simulink model "spherical_5th_traj_ctc"  (R2020b)
settings: Solver=ode4  StartTime=0.0  StopTime=2  FixedStep=0.001  RelTol=1e-3
values from neighbouring files (symbols this model uses):
  theta_m0_from_IK = N * theta0_from_IK    [start_taskspace_quintic_timeseries.m]
  theta_mdot0_from_IK = N * theta_dot0_from_IK    [start_taskspace_quintic_timeseries.m]
settings Model: Creator=user  LastModifiedBy=user

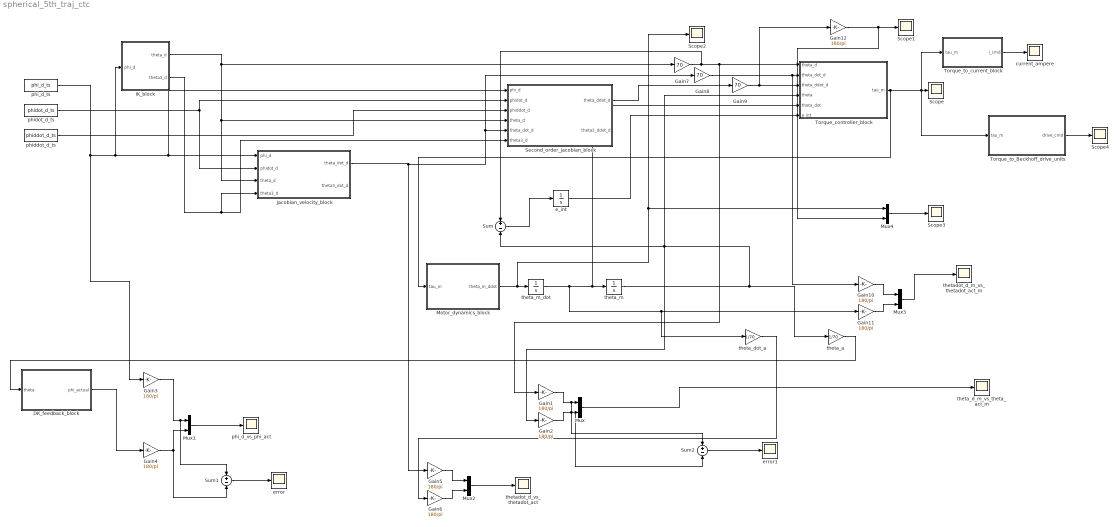
== system spherical_5th_traj_ctc ==
  DK_feedback_block : MATLAB Function  TreatAsAtomicUnit=on
  Gain{1..6,10..12} (9 alike) : Gain  Gain=180/pi
  Gain7 : Gain  Gain=70
  Gain8 : Gain  Gain=70
  Gain9 : Gain  Gain=70
  IK_block : MATLAB Function  TreatAsAtomicUnit=on
  Jacobian_velocity_block : MATLAB Function  TreatAsAtomicUnit=on
  Motor_dynamics_block : MATLAB Function  TreatAsAtomicUnit=on
  Mux{,1..4} (5 alike) : Mux  Inputs=2
  Scope{,1..4} (5 alike) : Scope
  Second_order_jacobian_block : MATLAB Function  TreatAsAtomicUnit=on
  Sum : Sum  Inputs=+-
  Sum1 : Sum  Inputs=+-
  Sum2 : Sum  Inputs=+-
  Torque_controller_block : MATLAB Function  TreatAsAtomicUnit=on
  Torque_to_Beckhoff_drive_units : MATLAB Function  TreatAsAtomicUnit=on
  Torque_to_current_block : MATLAB Function  TreatAsAtomicUnit=on
  current_ampere : Scope
  e_int : Integrator  InitialCondition=[0;0]
  error : Scope
  error1 : Scope
  phi_d_ts : FromWorkspace  VariableName=phi_d_ts  SampleTime=-1  OutputAfterFinalValue=Holding final value
  phi_d_vs_phi_act : Scope
  phiddot_d_ts : FromWorkspace  VariableName=phiddot_d_ts  SampleTime=-1  OutputAfterFinalValue=Holding final value
  phidot_d_ts : FromWorkspace  VariableName=phidot_d_ts  SampleTime=-1  OutputAfterFinalValue=Holding final value
  theta_a : Gain  Gain=1/70
  theta_d_m_vs_theta_act_m : Scope
  theta_dot_a : Gain  Gain=1/70
  theta_m : Integrator  InitialCondition=theta_m0_from_IK
  theta_m_dot : Integrator  InitialCondition=theta_mdot0_from_IK
  thetadot_d_m_vs_thetadot_act_m : Scope
  thetadot_d_vs_thetadot_act : Scope
  wires:
  phi_d_ts/1 -> Gain3/1, Jacobian_velocity_block/1(phi_d), Second_order_jacobian_block/1(phi_d), IK_block/1(phi_d)
  phidot_d_ts/1 -> Jacobian_velocity_block/2(phidot_d), Second_order_jacobian_block/2(phidot_d)
  IK_block/1(theta_d) -> Jacobian_velocity_block/3(theta_d), Second_order_jacobian_block/4(theta_d), Gain7/1
  IK_block/2(theta3_d) -> Jacobian_velocity_block/4(theta3_d), Second_order_jacobian_block/6(theta3_d)
  phiddot_d_ts/1 -> Second_order_jacobian_block/3(phiddot_d)
  Jacobian_velocity_block/1(theta_dot_d) -> Gain8/1, Second_order_jacobian_block/5(theta_dot_d), Gain5/1
  Second_order_jacobian_block/1(theta_ddot_d) -> Gain9/1
  Torque_controller_block/1(tau_m) -> Motor_dynamics_block/1(tau_m), Torque_to_current_block/1(tau_m), Scope/1, Torque_to_Beckhoff_drive_units/1(tau_m)
  Sum/1 -> e_int/1
  Mux/1 -> theta_d_m_vs_theta_act_m/1
  Gain3/1 -> Sum1/1, Mux1/1
  Mux1/1 -> phi_d_vs_phi_act/1
  Gain4/1 -> Sum1/2, Mux1/2
  DK_feedback_block/1(phi_actual) -> Gain4/1
  Gain5/1 -> Mux2/1
  Mux2/1 -> thetadot_d_vs_thetadot_act/1
  Gain6/1 -> Mux2/2
  Sum1/1 -> error/1
  Gain2/1 -> Sum2/2, Mux/2
  Sum2/1 -> error1/1
  Gain1/1 -> Sum2/1, Mux/1
  Gain7/1 -> Torque_controller_block/1(theta_d), Gain1/1, Sum/1
  Gain8/1 -> Gain10/1, Torque_controller_block/2(theta_dot_d)
  theta_m_dot/1 -> theta_m/1, Torque_controller_block/5(theta_dot), theta_dot_a/1, Gain11/1
  e_int/1 -> Torque_controller_block/6(e_int)
  theta_m/1 -> theta_a/1, Torque_controller_block/4(theta), Sum/2, Gain2/1
  theta_a/1 -> DK_feedback_block/1(theta)
  theta_dot_a/1 -> Gain6/1
  Gain11/1 -> Mux3/2
  Gain10/1 -> Mux3/1
  Mux3/1 -> thetadot_d_m_vs_thetadot_act_m/1
  Gain9/1 -> Torque_controller_block/3(theta_ddot_d), Gain12/1
  Motor_dynamics_block/1(theta_m_ddot) -> Mux4/1, Scope2/1, theta_m_dot/1
  Gain12/1 -> Mux4/2, Scope1/1
  Torque_to_current_block/1(i_cmd) -> current_ampere/1
  Mux4/1 -> Scope3/1
  Torque_to_Beckhoff_drive_units/1(drive_cmd) -> Scope4/1

== matlab function spherical_5th_traj_ctc/Jacobian_velocity_block ==
  data: phi_d input double size=[2 1]; theta_dot_d output double size=[2 1]; phidot_d input double size=[2 1]; theta_d input double size=[2 1]; theta3_d input double size=[1 1]; theta3_dot_d output double size=[1 1]
function [theta_dot_d, theta3_dot_d] = Jacobian_velocity_block(phi_d, phidot_d, theta_d, theta3_d)


deg = pi/180;

%% Robot parameters
alpha0 = pi/2;
alpha1 = pi/2;
alpha2 = pi/2;
alpha3 = pi/2;

beta1 = 0;
beta2 = 75*deg;

%% Inputs
theta1 = theta_d(1);
theta2 = theta_d(2);
theta3 = theta3_d;

phi1 = phi_d(1);

%% Rotation matrices
Rot_Y = @(a)[cos(a), 0, sin(a);
             0,      1, 0;
            -sin(a), 0, cos(a)];

Rot_DH = @(a,t)[cos(t), -sin(t)*cos(a),  sin(t)*sin(a);
                sin(t),  cos(t)*cos(a), -cos(t)*sin(a);
                0,       sin(a),         cos(a)];

%% Unit vectors
e1 = [0;0;1];
e2 = [1;0;0];

e33 = [0;0;1];
e44 = [0;0;1];
e55 = [0;0;1];

%% End-effector vector in frame 5
v5 = [sin(beta2);
      sin(beta1)*cos(beta2);
      cos(beta1)*cos(beta2)];

v5 = v5 / norm(v5);

%% Transformations
Q0 = Rot_Y(alpha0);
Q1 = Rot_DH(alpha1, theta1);
Q2 = Rot_DH(alpha2, theta2);
Q3 = Rot_DH(alpha3, theta3);

%% Vectors in frame 1
e3 = Q1 * e33;
e4 = Q0 * Q2 * e44;

e5 = Q1 * Q3 * e55;
e5 = e5 / norm(e5);

v1 = Q1 * Q3 * v5;
v1 = v1 / norm(v1);

%% Angular velocity mapping
% omega_1 = S * phidot
S = [0,  sin(phi1);
     0, -cos(phi1);
     1,  0];

%% Jacobian terms
k11 = dot(v1, cross(e1, e3));
k22 = dot(e5, cross(e2, e4));

J0 = [cross(e3, v1).';
      cross(e4, e5).'];

J = J0 * S;

%% Avoid division by exact zero
epsK = 1e-8;

if abs(k11) < epsK
    k11 = sign_or_one(k11) * epsK;
end

if abs(k22) < epsK
    k22 = sign_or_one(k22) * epsK;
end

%% Velocity mapping
% K * theta_dot = J * phi_dot
theta1_dot = (J(1,:) * phidot_d) / k11;
theta2_dot = (J(2,:) * phidot_d) / k22;

theta_dot_d = [theta1_dot;
               theta2_dot];

%% Passive joint velocity
omega = S * phidot_d;

theta3_dot_d = dot(e3, omega);

end

function y = sign_or_one(x)

if x >= 0
    y = 1;
else
    y = -1;
end

end

== matlab function spherical_5th_traj_ctc/IK_block ==
  settings: updateMethod=DISCRETE
  data: phi_d input double size=[2 1]; theta_d output double size=[2 1]; theta3_d output double size=[1 1]
function [theta_d, theta3_d] = IK_block(phi_d)


deg = pi/180;

alpha0 = pi/2;
alpha1 = pi/2;
alpha2 = pi/2;
alpha3 = pi/2;
alpha4 = pi/2;

beta1 = 0;
beta2 = 75*deg;

theta3_ref = 15*deg;

tol = 1e-9;
tolPhi1 = 1e-8;

phi1 = phi_d(1);
phi2 = phi_d(2);

d_des = direction_from_orientation(phi1, phi2);

persistent theta_prev initialized

if isempty(initialized)
    theta_prev = [0; 0; theta3_ref];
    initialized = true;
end

sols = zeros(6,3);
valid = false(6,1);
idx = 0;

%% Special DK-consistent branch
% phi1 = 0 -> theta1 = 0, theta2 = phi2, theta3 = 15 + theta2

if abs(phi1) < tolPhi1

    theta1 = 0;
    theta2 = phi2;
    theta3 = theta3_ref + theta2;

    d_check = FK_direction(theta1, theta3, beta1, beta2, alpha1, alpha3);
    err = norm(d_check - d_des);

    if err < 1e-6
        idx = idx + 1;
        sols(idx,:) = [theta1, theta2, theta3];
        valid(idx) = true;
    end
end

%% Normal IK branches

Rot_Y = @(a)[cos(a) 0 sin(a);
             0      1 0;
            -sin(a) 0 cos(a)];

Rot_DH = @(a,t)[cos(t), -sin(t)*cos(a),  sin(t)*sin(a);
                sin(t),  cos(t)*cos(a), -cos(t)*sin(a);
                0,       sin(a),         cos(a)];

Q0 = Rot_Y(alpha0);

e11 = [0;0;1];
e44 = [0;0;1];

v5 = [sin(beta2);
      sin(beta1)*cos(beta2);
      cos(beta1)*cos(beta2)];

v5 = v5 / norm(v5);

v = [ d_des(2);
     -d_des(1);
      d_des(3)];

v = v / norm(v);

vx = v(1);
vy = v(2);

b = sin(beta1)*cos(beta2);
R = sqrt(vx^2 + vy^2);

if R > tol && abs(b) <= R + tol

    ratio = clamp(b/R, -1, 1);
    psi = atan2(vy, vx);

    theta1_list = zeros(2,1);
    theta1_list(1) = wrapToPiLocal(psi + asin(ratio));
    theta1_list(2) = wrapToPiLocal(psi + pi - asin(ratio));

    a = sin(beta2);
    c = cos(beta1)*cos(beta2);

    for i = 1:2

        theta1 = theta1_list(i);
        Q1 = Rot_DH(alpha1, theta1);

        A = Q1.' * v;

        denom = a^2 + c^2;

        if denom > tol

            cos3 = (a*A(1) - c*A(2)) / denom;
            sin3 = (c*A(1) + a*A(2)) / denom;

            cos3 = clamp(cos3, -1, 1);
            sin3 = clamp(sin3, -1, 1);

            theta3 = wrapToPiLocal(atan2(sin3, cos3));
            Q3 = Rot_DH(alpha3, theta3);

            if norm(Q1*Q3*v5 - v) < 1e-6

                u = Q1 * Q3 * e11;
                u = u / norm(u);

                C = cos(alpha4);

                A2 = -u(3);
                B2 = -u(2);

                R2 = sqrt(A2^2 + B2^2);

                if R2 > tol && abs(C) <= R2 + tol

                    ratio2 = clamp(C/R2, -1, 1);
                    delta = atan2(B2, A2);

                    theta2_a = wrapToPiLocal(asin(ratio2) - delta);
                    theta2_b = wrapToPiLocal(pi - asin(ratio2) - delta);

                    theta2_list = [theta2_a; theta2_b];

                    for m = 1:2

                        theta2 = theta2_list(m);
                        Q2 = Rot_DH(alpha2, theta2);

                        e41 = Q0 * Q2 * e44;

                        constraint_error = dot(u,e41) - cos(alpha4);

                        if abs(constraint_error) < 1e-6

                            d_check = FK_direction(theta1, theta3, beta1, beta2, alpha1, alpha3);
                            err = norm(d_check - d_des);

                            if err < 1e-6 && idx < 6
                                idx = idx + 1;
                                sols(idx,:) = [theta1, theta2, theta3];
                                valid(idx) = true;
                            end
                        end
                    end
                end
            end
        end
    end
end

%% Choose solution closest to previous joint state

bestCost = 1e9;
bestTheta = theta_prev;

for k = 1:6

    if valid(k)

        theta_k = sols(k,:).';

        cost = norm(wrapToPiVec(theta_k - theta_prev));

        if cost < bestCost
            bestCost = cost;
            bestTheta = theta_k;
        end
    end
end

theta_prev = bestTheta;

theta_d = [bestTheta(1); bestTheta(2)];
theta3_d = bestTheta(3);

end

%% ============================================================
% LOCAL FUNCTIONS
%% ============================================================

function d = direction_from_orientation(phi1, phi2)

d = [-cos(phi2)*sin(phi1);
      cos(phi2)*cos(phi1);
      sin(phi2)];

d = d / norm(d);
end

function d = FK_direction(theta1, theta3, beta1, beta2, alpha1, alpha3)

Rot_DH = @(a,t)[cos(t), -sin(t)*cos(a),  sin(t)*sin(a);
                sin(t),  cos(t)*cos(a), -cos(t)*sin(a);
                0,       sin(a),         cos(a)];

Q1 = Rot_DH(alpha1, theta1);
Q3 = Rot_DH(alpha3, theta3);

v5 = [sin(beta2);
      sin(beta1)*cos(beta2);
      cos(beta1)*cos(beta2)];

v5 = v5 / norm(v5);

v1 = Q1 * Q3 * v5;
v1 = v1 / norm(v1);

d = [-v1(2);
      v1(1);
      v1(3)];

d = d / norm(d);
end

function x = clamp(x, lo, hi)

x = min(max(x, lo), hi);
end

function a = wrapToPiLocal(a)

a = atan2(sin(a), cos(a));
end

function y = wrapToPiVec(x)

y = zeros(size(x));

for i = 1:length(x)
    y(i) = atan2(sin(x(i)), cos(x(i)));
end
end

== matlab function spherical_5th_traj_ctc/Second_order_jacobian_block ==
  data: phi_d input double size=[2 1]; theta_ddot_d output double size=[2 1]; phidot_d input double size=[2 1]; phiddot_d input double size=[2 1]; theta_d input double size=[2 1]; theta_dot_d input double size=[2 1]; theta3_d input double size=[1 1]; theta3_ddot_d output double size=[1 1]
function [theta_ddot_d, theta3_ddot_d] = Second_order_jacobian_block(phi_d, phidot_d, phiddot_d, theta_d, theta_dot_d, theta3_d)


deg = pi/180;

alpha0 = pi/2;
alpha1 = pi/2;
alpha2 = pi/2;
alpha3 = pi/2;

beta1 = 0;
beta2 = 75*deg;

theta1 = theta_d(1);
theta2 = theta_d(2);
theta3 = theta3_d;

theta1_dot = theta_dot_d(1);
theta2_dot = theta_dot_d(2);

phi1 = phi_d(1);

Rot_Y = @(a)[cos(a), 0, sin(a);
             0,      1, 0;
            -sin(a), 0, cos(a)];

Rot_DH = @(a,t)[cos(t), -sin(t)*cos(a),  sin(t)*sin(a);
                sin(t),  cos(t)*cos(a), -cos(t)*sin(a);
                0,       sin(a),         cos(a)];

e1 = [0;0;1];
e2 = [1;0;0];

e33 = [0;0;1];
e44 = [0;0;1];
e55 = [0;0;1];

v5 = [sin(beta2);
      sin(beta1)*cos(beta2);
      cos(beta1)*cos(beta2)];

v5 = v5 / norm(v5);

Q0 = Rot_Y(alpha0);
Q1 = Rot_DH(alpha1, theta1);
Q2 = Rot_DH(alpha2, theta2);
Q3 = Rot_DH(alpha3, theta3);

e3 = Q1 * e33;

e4 = Q0 * Q2 * e44;

e5 = Q1 * Q3 * e55;
e5 = e5 / norm(e5);

v1 = Q1 * Q3 * v5;
v1 = v1 / norm(v1);


S = [0,  sin(phi1);
     0, -cos(phi1);
     1,  0];

Sdot = [0,  cos(phi1)*phidot_d(1);
        0,  sin(phi1)*phidot_d(1);
        0,  0];

omega = S * phidot_d;

omega_dot = S * phiddot_d + Sdot * phidot_d;


e3_dot = theta1_dot * cross(e1, e3);

e4_dot = theta2_dot * cross(e2, e4);

v1_dot = cross(omega, v1);

e5_dot = cross(omega, e5);

% e3_ddot = theta1_ddot*(e1 x e3) + theta1_dot*(e1 x e3_dot)
e3_ddot_known = theta1_dot * cross(e1, e3_dot);

% e4_ddot = theta2_ddot*(e2 x e4) + theta2_dot*(e2 x e4_dot)
e4_ddot_known = theta2_dot * cross(e2, e4_dot);

% v1_ddot = omega_dot x v1 + omega x v1_dot
v1_ddot = cross(omega_dot, v1) + cross(omega, v1_dot);

% e5_ddot = omega_dot x e5 + omega x e5_dot
e5_ddot = cross(omega_dot, e5) + cross(omega, e5_dot);

%% ============================================================
% Acceleration constraint 1
%% ============================================================
%
% C1 = e3 . v1 = constant
%
% C1_ddot =
% e3_ddot . v1 + 2 e3_dot . v1_dot + e3 . v1_ddot = 0
%
% Solve for theta1_ddot

den1 = dot(v1, cross(e1, e3));

num1 = dot(e3_ddot_known, v1) + 2 * dot(e3_dot, v1_dot)+ dot(e3, v1_ddot);

epsD = 1e-8;

if abs(den1) < epsD
    den1 = sign_or_one(den1) * epsD;
end

theta1_ddot = -num1 / den1;

%% ============================================================
% Acceleration constraint 2
%% ============================================================
%
% C2 = e4 . e5 = constant
%
% C2_ddot =
% e4_ddot . e5 + 2 e4_dot . e5_dot + e4 . e5_ddot = 0
%
% Solve for theta2_ddot

den2 = dot(e5, cross(e2, e4));

num2 = dot(e4_ddot_known, e5) + 2 * dot(e4_dot, e5_dot)+ dot(e4, e5_ddot);

if abs(den2) < epsD
    den2 = sign_or_one(den2) * epsD;
end

theta2_ddot = -num2 / den2;

theta_ddot_d = [theta1_ddot;
                theta2_ddot];

%% ============================================================
% Passive joint acceleration
%% ============================================================
%
% omega_dot = theta1_ddot*e1 + theta3_ddot*e3 + theta3_dot*e3_dot
%
% We approximate from platform angular acceleration:
%
% theta3_ddot = e3 . omega_dot

theta3_ddot_d = dot(e3, omega_dot);

end

function y = sign_or_one(x)

if x >= 0
    y = 1;
else
    y = -1;
end

end

== matlab function spherical_5th_traj_ctc/Torque_controller_block ==
  data: theta_d input double size=[2 1]; tau_m output double size=[2 1]; theta_dot_d input double size=[2 1]; theta_ddot_d input double size=[2 1]; theta input double size=[2 1]; theta_dot input double size=[2 1]; e_int input double size=[2 1]
function tau_m = Torque_controller_block(theta_d, theta_dot_d, theta_ddot_d, theta, theta_dot, e_int)

J1 = 62e-6;
J2 = 62e-6;    

%% Controller gains from Beckhoff parameter file

Wc_B = 150.0;
Wn_B = 2*Wc_B;

Ki_B = Wn_B^3;
Kp_B = 3*Wn_B^2;
Kv_B = 3*Wn_B;

Kp1 = Kp_B;
Kp2 = Kp_B;

Kd1 = Kv_B;
Kd2 = Kv_B;

Ki1 = Ki_B;
Ki2 = Ki_B;


e1 = theta_d(1) - theta(1);
e2 = theta_d(2) - theta(2);

ed1 = theta_dot_d(1) - theta_dot(1);
ed2 = theta_dot_d(2) - theta_dot(2);

ei1 = e_int(1);
ei2 = e_int(2);


v1 = theta_ddot_d(1) + Kd1*ed1 + Kp1*e1 + Ki1*ei1;
v2 = theta_ddot_d(2) + Kd2*ed2 + Kp2*e2 + Ki2*ei2;

tau1 = J1 * v1;
tau2 = J2 * v2;

%% Torque saturation
tau_max = 1.0;    % Nm

if tau1 > tau_max
    tau1 = tau_max;
elseif tau1 < -tau_max
    tau1 = -tau_max;
end

if tau2 > tau_max
    tau2 = tau_max;
elseif tau2 < -tau_max
    tau2 = -tau_max;
end

tau_m = [tau1;
       tau2];

end

== matlab function spherical_5th_traj_ctc/DK_feedback_block ==
  data: theta input double size=[2 1]; phi_actual output double size=[2 1]
function phi_actual = DK_feedback_block(theta)

deg = pi/180;

%% Robot parameters
alpha0 = pi/2;
alpha1 = pi/2;
alpha2 = pi/2;
alpha3 = pi/2;

beta1 = 0;
beta2 = 75*deg;

theta3_home = 15*deg;

tolTheta  = 1e-10;
tolTheta1 = 1e-8;
tolCross  = 1e-10;

theta1 = theta(1);
theta2 = theta(2);

%% Rotation matrices
Rot_Y = @(a)[cos(a), 0, sin(a);
             0,      1, 0;
            -sin(a), 0, cos(a)];

Rot_DH = @(a,t)[cos(t), -sin(t)*cos(a),  sin(t)*sin(a);
                sin(t),  cos(t)*cos(a), -cos(t)*sin(a);
                0,       sin(a),         cos(a)];

%% Unit vectors
e33 = [0;0;1];
e44 = [0;0;1];
e55 = [0;0;1];

%% v5
v5 = [sin(beta2);
      sin(beta1)*cos(beta2);
      cos(beta1)*cos(beta2)];

v5 = v5 / norm(v5);

%% Transformations
Q0 = Rot_Y(alpha0);
Q1 = Rot_DH(alpha1, theta1);
Q2 = Rot_DH(alpha2, theta2);

e3 = Q1 * e33;
e4 = Q0 * Q2 * e44;

cross_e = cross(e3, e4);
cross_norm = norm(cross_e);

%% DK branch logic
if abs(theta1) < tolTheta1

    % Physical theta1 = 0 branch
    theta3 = theta3_home + theta2;

elseif cross_norm < tolCross

    % Fallback at true cross-product singularity
    theta3 = theta3_home;

else

    % General DK branch
    u_plus  =  cross_e / cross_norm;
    u_minus = -cross_e / cross_norm;

    theta3_plus  = theta3_from_u(u_plus,  theta1, tolTheta);
    theta3_minus = theta3_from_u(u_minus, theta1, tolTheta);

    err_plus  = abs(wrapToPiLocal(theta3_plus  - theta3_home));
    err_minus = abs(wrapToPiLocal(theta3_minus - theta3_home));

    if err_plus <= err_minus
        theta3 = theta3_plus;
    else
        theta3 = theta3_minus;
    end
end

%% Output direction
Q3 = Rot_DH(alpha3, theta3);

v1 = Q1 * Q3 * v5;
v1 = v1 / norm(v1);

d = [-v1(2);
      v1(1);
      v1(3)];

d = d / norm(d);

phi1 = atan2(-d(1), d(2));
phi2 = asin(clamp(d(3), -1, 1));

phi_actual = [phi1;
              phi2];

end

%% ============================================================
% Helper functions
%% ============================================================

function theta3 = theta3_from_u(u, theta1, tol)

ux = u(1);
uy = u(2);
uz = u(3);

if abs(cos(theta1)) > abs(sin(theta1))
    sin_theta3 = ux / cos(theta1);
else
    if abs(sin(theta1)) < tol
        sin_theta3 = 0;
    else
        sin_theta3 = uy / sin(theta1);
    end
end

cos_theta3 = -uz;

sin_theta3 = clamp(sin_theta3, -1, 1);
cos_theta3 = clamp(cos_theta3, -1, 1);

theta3 = atan2(sin_theta3, cos_theta3);

end

function x = clamp(x, lo, hi)

x = min(max(x, lo), hi);

end

function a = wrapToPiLocal(a)

a = atan2(sin(a), cos(a));

end

== matlab function spherical_5th_traj_ctc/Motor_dynamics_block ==
  data: tau_m input double size=[2 1]; theta_m_ddot output double size=[2 1]
function theta_m_ddot = Motor_dynamics_block(tau_m)
J1 = 62e-6;
J2 = 62e-6;
theta1_ddot = tau_m(1) / J1;
theta2_ddot = tau_m(2) / J2;

theta_m_ddot = [theta1_ddot;
              theta2_ddot];

end

== matlab function spherical_5th_traj_ctc/Torque_to_current_block ==
  data: tau_m input; i_cmd output
function i_cmd = Torque_to_current_block(tau_m)

Kt = 0.54;          % Nm/A, Beckhoff motor torque constant
tau_max = 1.0;     % Nm, 

i_max = tau_max / Kt;

i1 = tau_m(1) / Kt;
i2 = tau_m(2) / Kt;

% Current saturation
if i1 > i_max
    i1 = i_max;
elseif i1 < -i_max
    i1 = -i_max;
end

if i2 > i_max
    i2 = i_max;
elseif i2 < -i_max
    i2 = -i_max;
end

i_cmd = [i1; i2];

end

== matlab function spherical_5th_traj_ctc/Torque_to_Beckhoff_drive_units ==
  data: tau_m input; drive_cmd output
function drive_cmd = Torque_to_Beckhoff_drive_units(tau_m)
%#codegen
% Converts motor torque command [Nm] into Beckhoff drive torque units

% Beckhoff motor/drive constants
Kt = 0.54;             % Nm/A
peak_current = 4.4;    % A

% Conservative motor torque limit
tau_max = 1.0;         % Nm

% Drive scaling from robot.h:
% UNITS_TORQUE_B = 1000/(PEAK_CURRENT_B*KT_B)
units_torque = 1000 / (peak_current * Kt);

% Saturate torque first
tau1 = tau_m(1);
tau2 = tau_m(2);

if tau1 > tau_max
    tau1 = tau_max;
elseif tau1 < -tau_max
    tau1 = -tau_max;
end

if tau2 > tau_max
    tau2 = tau_max;
elseif tau2 < -tau_max
    tau2 = -tau_max;
end

% Convert Nm to drive command units
u1 = tau1 * units_torque;
u2 = tau2 * units_torque;

drive_cmd = [u1; u2];

end
